simulink model "rtwdemo_switchsl"  (Simulink 7.1)
settings: Solver=FixedStepDiscrete  StartTime=0.0  StopTime=10.0  FixedStep=.01  RelTol=1e-3
settings Model: Creator=ajayaram  LastModifiedBy=ajayaram
settings SolverCC: AutoInsertRateTranBlk=on
settings DataIOCC: SaveOutput=off  SaveTime=off
settings OptimizationCC: InlineParams=on  InlineInvariantSignals=on  EnforceIntegerDowncast=off  StateBitsets=on  DataBitsets=on  UseTempVars=on  OptimizeModelRefInitCode=on  LifeSpan=1
settings DebuggingCC: SaveWithParameterizedLinksMsg=none
settings RTWCC: SystemTargetFile=ert.tlc  GenCodeOnly=on  GenerateMakefile=off  TemplateMakefile=ert_default_tmf  Description=Real-Time Workshop Embedded Coder (no auto configuration)  GenerateReport=on  RTWVerbose=off  ProcessScript=ert_make_rtw_hook  IncludeHyperlinkInReport=on  LaunchReport=on
settings CodeAppCC: GenerateComments=off  IgnoreCustomStorageClasses=off  CustomSymbolStrGlobalVar=rt$N$M  CustomSymbolStrType=$N$M  CustomSymbolStrFcn=$N$M$F  CustomSymbolStrMacro=$N$M  SimulinkBlockComments=off
settings ERTTargetCC: GenerateSampleERTMain=on  SuppressErrorStatus=on  SupportAbsoluteTime=off  SupportNonFinite=off  SupportComplex=off  InlinedParameterPlacement=NonHierarchical  RootIOFormat=Structure reference  ERTCustomFileTemplate=example_file_process.tlc

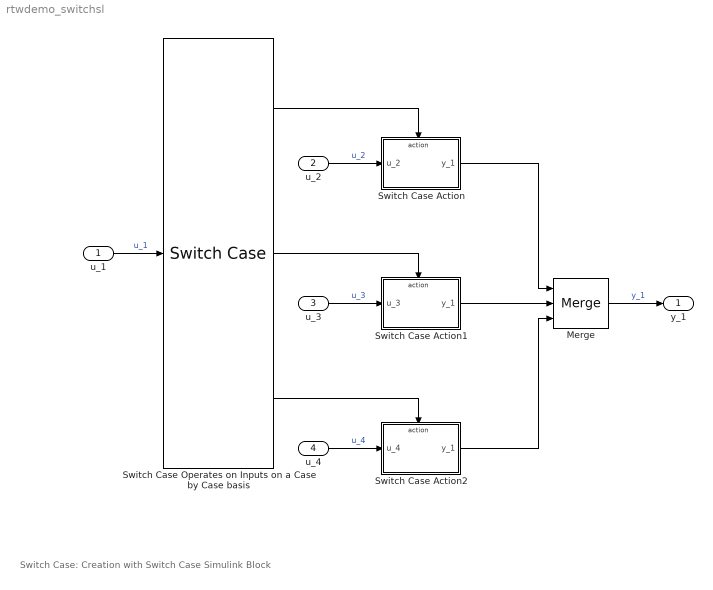
== system rtwdemo_switchsl ==
  note: Switch Case: Creation with
      | Switch Case Simulink Block
  u_1 : Inport  DataType=uint32  OutDataType=sfix(16)  OutScaling=2^0  OutDataTypeStr=uint32
  u_2 : Inport  Port=2  OutDataType=sfix(16)  OutScaling=2^0
  u_3 : Inport  Port=3  OutDataType=sfix(16)  OutScaling=2^0
  u_4 : Inport  Port=4  OutDataType=sfix(16)  OutScaling=2^0
  Merge : Merge  Inputs=3
  Switch Case Operates on Inputs on a Case by Case basis : SwitchCase  CaseConditions={2,3}
  Switch Case Action : Subsystem  TreatAsAtomicUnit=on
      settings: RTWSystemCode=Inline
  "Switch Case Action1 " : Subsystem  TreatAsAtomicUnit=on
      settings: RTWSystemCode=Inline
  Switch Case Action2 : Subsystem  TreatAsAtomicUnit=on
      settings: RTWSystemCode=Inline
  y_1 : Outport  OutDataType=sfix(16)  OutScaling=2^0
  wires:
  u_1/1 -> Switch Case Operates on Inputs on a Case by Case basis/1  "u_1"
  Switch Case Operates on Inputs on a Case by Case basis/1 -> Switch Case Action/Action
  Switch Case Operates on Inputs on a Case by Case basis/2 -> "Switch Case Action1 "/Action
  Switch Case Operates on Inputs on a Case by Case basis/3 -> Switch Case Action2/Action
  u_4/1 -> Switch Case Action2/1(u_4)  "u_4"
  u_3/1 -> "Switch Case Action1 "/1(u_3)  "u_3"
  u_2/1 -> Switch Case Action/1(u_2)  "u_2"
  Switch Case Action/1(y_1) -> Merge/1
  Switch Case Action2/1(y_1) -> Merge/3
  Merge/1 -> y_1/1  "y_1"
  "Switch Case Action1 "/1(y_1) -> Merge/2

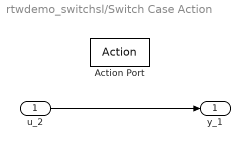
== system rtwdemo_switchsl/Switch Case Action ==
  u_2 : Inport  OutDataType=sfix(16)  OutScaling=2^0
  Action Port : ActionPort  ActionType=case
  y_1 : Outport  OutDataType=sfix(16)  OutScaling=2^0
  wires:
  u_2/1 -> y_1/1

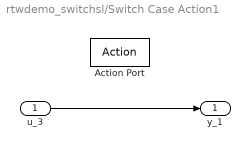
== system rtwdemo_switchsl/Switch Case Action1  ==
  u_3 : Inport  OutDataType=sfix(16)  OutScaling=2^0
  Action Port : ActionPort  ActionType=case
  y_1 : Outport  OutDataType=sfix(16)  OutScaling=2^0
  wires:
  u_3/1 -> y_1/1

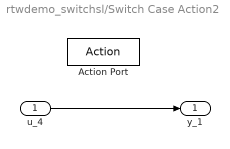
== system rtwdemo_switchsl/Switch Case Action2 ==
  u_4 : Inport  OutDataType=sfix(16)  OutScaling=2^0
  Action Port : ActionPort  ActionType=default
  y_1 : Outport  OutDataType=sfix(16)  OutScaling=2^0
  wires:
  u_4/1 -> y_1/1
